simulink model "Force_Models"  (R2017b)
settings: Solver=ode4  StartTime=0.0  StopTime=32  FixedStep=60  RelTol=1e-3
undefined symbols (not defined in the file or in its folder): AU, c, Cube, G, mu_s, SC, Sun
settings Model: Creator=hazr_sh  LastModifiedBy=hazr_sh

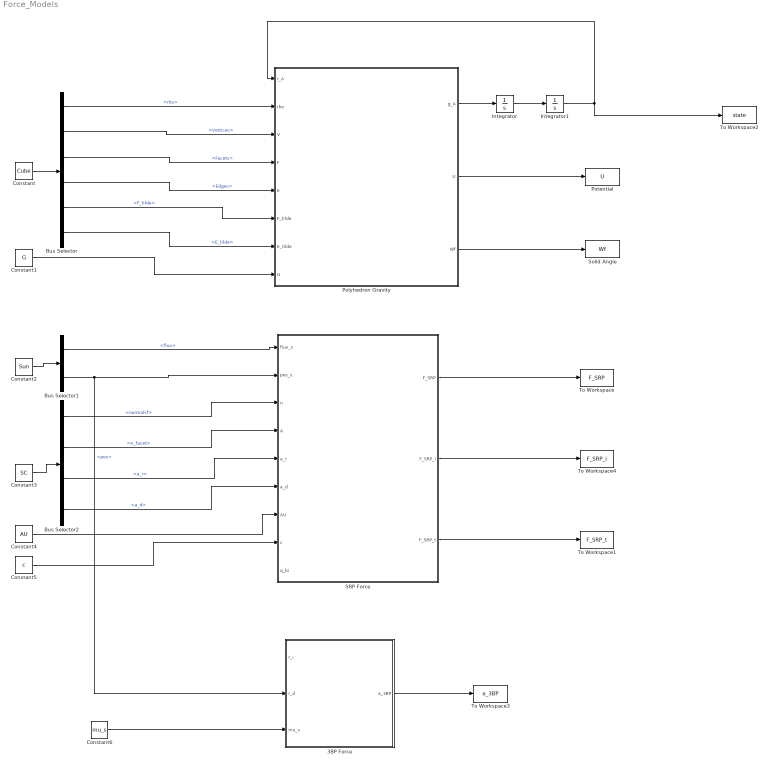
== system Force_Models ==
  3BP Force : MATLAB Function  TreatAsAtomicUnit=on
  Bus Selector : BusSelector  OutputSignals=rho,Polyhedron.Vertices,Polyhedron.Facets,Polyhedron.Edges,Polyhedron.F_tilde,Polyhedron.E_tilde
  Bus Selector1 : BusSelector  OutputSignals=flux,pos
  Bus Selector2 : BusSelector  OutputSignals=Polyhedron.normalsf,Polyhedron.A_facet,a_r,a_d
  Constant : Constant  Value=Cube  VectorParams1D=off  OutDataTypeStr=Bus: slBus1
  Constant1 : Constant  Value=G
  Constant2 : Constant  Value=Sun  VectorParams1D=off  OutDataTypeStr=Bus: slBus2
  Constant3 : Constant  Value=SC  VectorParams1D=off  OutDataTypeStr=Bus: slBus3
  Constant4 : Constant  Value=AU
  Constant5 : Constant  Value=c
  Constant6 : Constant  Value=mu_s
  Integrator : Integrator  InitialCondition=SC.v_init
  Integrator1 : Integrator  InitialCondition=SC.x_init
  Polyhedron Gravity : MATLAB Function  TreatAsAtomicUnit=on
  Potential : ToWorkspace  VariableName=U  SaveFormat=Timeseries  SampleTime=-1
  SRP Force : MATLAB Function  TreatAsAtomicUnit=on
  Solid Angle : ToWorkspace  VariableName=Wf  SaveFormat=Timeseries  SampleTime=-1
  To Workspace : ToWorkspace  VariableName=F_SRP  SampleTime=-1
      settings: Save2DSignal=2-D array (concatenate along first dimension)
  To Workspace1 : ToWorkspace  VariableName=F_SRP_t  SampleTime=-1
      settings: Save2DSignal=2-D array (concatenate along first dimension)
  To Workspace2 : ToWorkspace  VariableName=state  SampleTime=-1
  To Workspace3 : ToWorkspace  VariableName=a_3BP  SampleTime=-1
      settings: Save2DSignal=2-D array (concatenate along first dimension)
  To Workspace4 : ToWorkspace  VariableName=F_SRP_i  SampleTime=-1
      settings: Save2DSignal=2-D array (concatenate along first dimension)
  wires:
  Constant2/1 -> Bus Selector1/1
  Bus Selector1/1 -> SRP Force/1(flux_s)  "<flux>"
  Constant3/1 -> Bus Selector2/1
  Bus Selector1/2 -> 3BP Force/2(r_d), SRP Force/2(pos_s)  "<pos>"
  Bus Selector2/1 -> SRP Force/3(n)  "<normalsf>"
  Bus Selector2/2 -> SRP Force/4(A)  "<A_facet>"
  Bus Selector2/3 -> SRP Force/5(a_r)  "<a_r>"
  Bus Selector2/4 -> SRP Force/6(a_d)  "<a_d>"
  Constant4/1 -> SRP Force/7(AU)
  Constant5/1 -> SRP Force/8(c)
  SRP Force/1(F_SRP) -> To Workspace/1
  SRP Force/3(F_SRP_t) -> To Workspace1/1
  Constant/1 -> Bus Selector/1
  Bus Selector/1 -> Polyhedron Gravity/2(rho)  "<rho>"
  Bus Selector/3 -> Polyhedron Gravity/4(F)  "<Facets>"
  Bus Selector/4 -> Polyhedron Gravity/5(E)  "<Edges>"
  Bus Selector/5 -> Polyhedron Gravity/6(F_tilde)  "<F_tilde>"
  Bus Selector/6 -> Polyhedron Gravity/7(E_tilde)  "<E_tilde>"
  Integrator/1 -> Integrator1/1
  Constant1/1 -> Polyhedron Gravity/8(G)
  Polyhedron Gravity/2(U) -> Potential/1
  Polyhedron Gravity/3(Wf) -> Solid Angle/1
  Polyhedron Gravity/1(g_A) -> Integrator/1
  Integrator1/1 -> To Workspace2/1, Polyhedron Gravity/1(r_A)
  Bus Selector/2 -> Polyhedron Gravity/3(V)  "<Vertices>"
  Constant6/1 -> 3BP Force/3(mu_s)
  3BP Force/1(a_3BP) -> To Workspace3/1
  SRP Force/2(F_SRP_i) -> To Workspace4/1
  ? -> SRP Force/9(q_bi)
  ? -> 3BP Force/1(r_i)

== matlab function Force_Models/SRP Force ==
  data: flux_s input; pos_s input; n input; A input; a_r input; a_d input; AU input; c input; F_SRP output; F_SRP_i output; F_SRP_t output; q_bi input
function [F_SRP,F_SRP_i,F_SRP_t]   = F_SRP(flux_s,pos_s,n,A,a_r,a_d,AU,c,q_bi)

e = pos_s(1,1:3)/norm(pos_s(1,1:3));
P = flux_s/(norm(pos_s(1,1:3)/AU)^2*c);

F_SRP = zeros(size(n,1),3); 
for i=1:1:size(n,1)
    
    co = dot(n(i,1:3),e(1,1:3),2);

    if i<=12
        F = -P*A(i,:)*co.*((2*(a_d(1,1)/3 + a_r(1,1)*co))'.*n(i,1:3) + (1-a_r(1,1))'.*e);
        F_SRP(i,:) = F;
    else
        F = -P*A(i,:)*co.*((2*(a_d(1,2)/3 + a_r(1,2)*co))'.*n(i,1:3) + (1-a_r(1,2))'.*e);
        F_SRP(i,:) = F;
    end
    
    
end
% 
F_SRP_i = cross_quat(q_bi,cross_quat([F_SRP 0]',conj_quat(q_bi)));
F_SRP_t = sum(F_SRP);

end

== matlab function Force_Models/Polyhedron Gravity ==
  data: r_A input; rho input; V input; F input; E input; F_tilde input; E_tilde input; g_A output; G input; U output; Wf output
function [g_A, U, Wf] = Poly_gravity(r_A,rho,V,F,E,F_tilde,E_tilde,G)
%% Function to calculate Cube gravity from Asteroid structure (from Get_Asteroid function)
%
% Inputs: r_A - position of a field point in Asteroid frame
%         Asteroid - Asteroid structure
%
% Outputs: g_A - gravitational acceleration in Asteroid frame
%          U - gravitational potential in Asteroid frame
%          Wf - THE solid angle, which shows whether the point is in or out
%               It can be used for stopping simulation if SC crashes

%% Initialization

Wf = 0;

Facets = [0 0 0]';
Edges = [0 0 0]';

U_edg = 0;
U_fac = 0;

S = r_A;

for j=1:1:size(E,1)
    
    % Calculate gravity due to edge potential
    
    R1 = V(E(j,1),:);    
    R2 = V(E(j,2),:);    

    Ri = R1'-S;
    ri = norm(Ri);
    
    Rj = R2'-S;
    rj = norm(Rj);
        
    Rij = Rj-Ri;
    eij = norm(Rij);

    Re1 =(Ri+Rj)/2;
   
    Le = log((ri+rj+eij)/(ri+rj-eij));
    
    if Le == Inf
     
        Le = 0;
     
    end
    
    Edges = (Le*E_tilde(:,:,j)*Re1)+Edges;
    U_edg = (Le*Re1'*E_tilde(:,:,j)*Re1)+U_edg;
    
end

 for i=1:1:(size(F,1))
    
    % Calculate gravity due to face potential
    
    R1 = V(F(i,1),:);    
    R2 = V(F(i,2),:);    
    R3 = V(F(i,3),:);
    

    Ri = R1'-S;
    ri = norm(Ri);
    
    Rj = R2'-S;
    rj = norm(Rj);
    
    Rk = R3'-S;
    rk = norm(Rk);
    
    
    wf = 2*atan2(dot(Ri, cross(Rj,Rk)),(ri*rj*rk+ri*dot(Rj,Rk)+rj*dot(Rk,Ri)+rk*dot(Ri,Rj)));
    
    Rf =(Ri+Rj+Rk)/3;

    U_fac = wf*Rf'*F_tilde(:,:,i)*Rf+U_fac;
    Facets = wf*F_tilde(:,:,i)*Rf+Facets;
    
    Wf = wf+Wf;
  
 end

g_A = G*rho*(-Edges+Facets);

U = 0.5*G*rho*(U_edg-U_fac);

end

== matlab function Force_Models/3BP Force ==
  data: r_i input; a_3BP output; r_d input; mu_s input
function a_3BP  = F_3BP(r_i,r_d,mu_s)

r_id = norm(r_d - r_i);
a_3BP = -G*m_s*(r_d-r_i/r_id^3 - r_d/norm(r_d)^3); 

end
